simulink model "4_MERGED_STATES"  (R2020a)
settings: Solver=FixedStepAuto  StartTime=0.0  StopTime=10.0  FixedStep=1e-3  RelTol=1e-3  EnableMultiTasking=on
undefined symbols (not defined in the file): D0, D1, D10, D11, D12, D13, D2, D3, D4, D5, D6, D7, D8, D9, PTA0, PTA1, PTA2, PTB23, PTB9, PTC16, PTC17, PTC2, PTC3, PTC4, PTD0, PTD1, PTD2, PTD3
libraries: frdmk64flib x14
settings Model: ExtModeTrigDuration=5  Creator=marry  LastModifiedBy=amnay
settings OptimizationCC: EnhancedBackFolding=on  PassReuseOutputArgsAs=Individual arguments  ZeroExternalMemoryAtStartup=off  ZeroInternalMemoryAtStartup=off  MaxStackSize=64  OptimizeBlockOrder=speed  DifferentSizesBufferReuse=on  OptimizationCustomize=off  EfficientTunableParamExpr=on
settings DebuggingCC: ParameterTunabilityLossMsg=error
settings HardwareCC: ProdBitPerPointer=32  ProdBitPerSizeT=32  ProdBitPerPtrDiffT=32  ProdLargestAtomicInteger=Long  ProdLargestAtomicFloat=Double  ProdWordSize=32  ProdHWDeviceType=ARM Compatible->ARM Cortex
settings SFSimCC: MATLABDynamicMemAlloc=off
settings RTWCC: SystemTargetFile=ert.tlc  HardwareBoard=NXP FRDM-K64F  TemplateMakefile=ert_default_tmf  Toolchain=GNU Tools for ARM Embedded Processors
settings CodeAppCC: ForceParamTrailComments=on  IgnoreCustomStorageClasses=off  OperatorAnnotations=on  SimulinkDataObjDesc=on  SFDataObjDesc=on  InsertBlockDesc=on

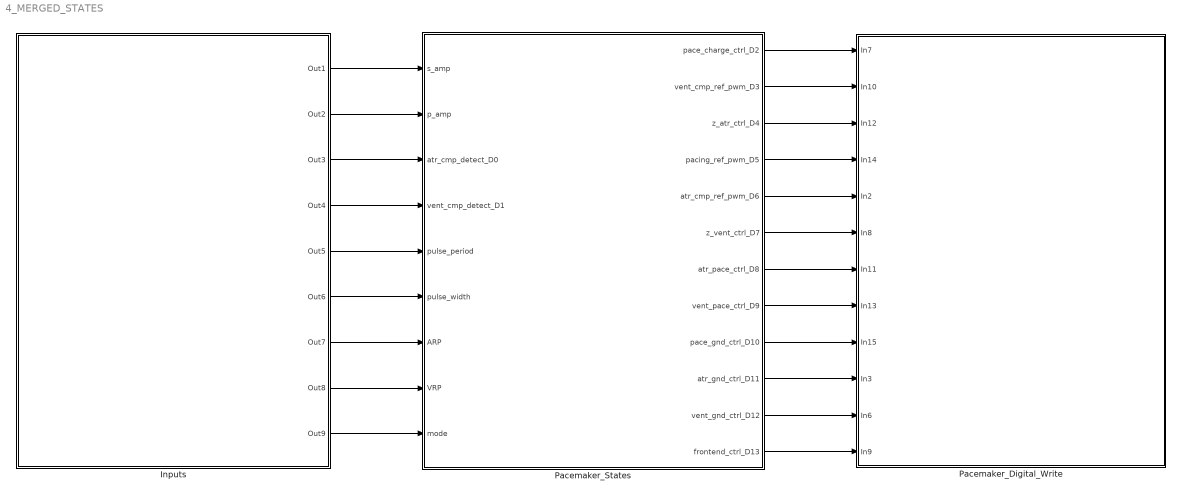
== system 4_MERGED_STATES ==
  Inputs : Subsystem
  Pacemaker_Digital_Write : Subsystem
  Pacemaker_States : Stateflow chart  TreatAsAtomicUnit=on
      settings: PortSchema="{\"entries\":[{\"content\":{\"sides\":[{\"content\":{\"connectorIds\":[\"In4\",\"In1\",\"In8\",\"In6\",\"In2\",\"In3\",\"In9\",\"In5\",\"In7\"]},\"type\":\"ConnectorPlacement.EquallySpacedRectSide\",\"uuid\":\"20680cc3-5670-44aa-8281-63eeb652eb93\"},{\"content\":{\"connectorIds\":[\"Out10\",\"Out7\",\"Out2\",\"Out8\",\"Out4\",\"Out1\",\"Out11\",\"Out3\",\"Out9\",\"Out5\",\"Out6\",\"Out12\"],\"side\":\"RIGHT\"},\"type\":\"ConnectorPlacement.EquallySpacedRectSide\",\"uuid\":\"3c751831-05e0-44c5-9153-358c656103ce\"},{\"content\":{\"connectorIds\":[],\"side\":\"TOP\"},\"type\":\"ConnectorPlacement.EquallySpacedRectSide\",\"uuid\":\"7efa84d7-9e28-4c8b-883e-bb8c609184af\"}]},\"type\":\"ConnectorPlacement.EquallySpacedConnector\",\"uuid\":\"9ce20c72-f6aa-4a08-b105-da4ff85e8db9\"}],\"packageUris\":[\"http://schema.mathworks.com/mf0/Connector/19700101\"],\"version\":\"1.0\"}"
  wires:
  Pacemaker_States/10(pace_charge_ctrl_D2) -> Pacemaker_Digital_Write/1(In7)
  Pacemaker_States/7(vent_cmp_ref_pwm_D3) -> Pacemaker_Digital_Write/2(In10)
  Pacemaker_States/8(pacing_ref_pwm_D5) -> Pacemaker_Digital_Write/4(In14)
  Pacemaker_States/2(z_atr_ctrl_D4) -> Pacemaker_Digital_Write/3(In12)
  Pacemaker_States/4(atr_cmp_ref_pwm_D6) -> Pacemaker_Digital_Write/5(In2)
  Pacemaker_States/1(z_vent_ctrl_D7) -> Pacemaker_Digital_Write/6(In8)
  Pacemaker_States/11(atr_pace_ctrl_D8) -> Pacemaker_Digital_Write/7(In11)
  Pacemaker_States/3(vent_pace_ctrl_D9) -> Pacemaker_Digital_Write/8(In13)
  Pacemaker_States/9(pace_gnd_ctrl_D10) -> Pacemaker_Digital_Write/9(In15)
  Pacemaker_States/5(atr_gnd_ctrl_D11) -> Pacemaker_Digital_Write/10(In3)
  Pacemaker_States/6(vent_gnd_ctrl_D12) -> Pacemaker_Digital_Write/11(In6)
  Pacemaker_States/12(frontend_ctrl_D13) -> Pacemaker_Digital_Write/12(In9)
  Inputs/1(Out1) -> Pacemaker_States/4(s_amp)
  Inputs/2(Out2) -> Pacemaker_States/1(p_amp)
  Inputs/3(Out3) -> Pacemaker_States/8(atr_cmp_detect_D0)
  Inputs/4(Out4) -> Pacemaker_States/6(vent_cmp_detect_D1)
  Inputs/5(Out5) -> Pacemaker_States/2(pulse_period)
  Inputs/6(Out6) -> Pacemaker_States/3(pulse_width)
  Inputs/7(Out7) -> Pacemaker_States/9(ARP)
  Inputs/8(Out8) -> Pacemaker_States/5(VRP)
  Inputs/9(Out9) -> Pacemaker_States/7(mode)

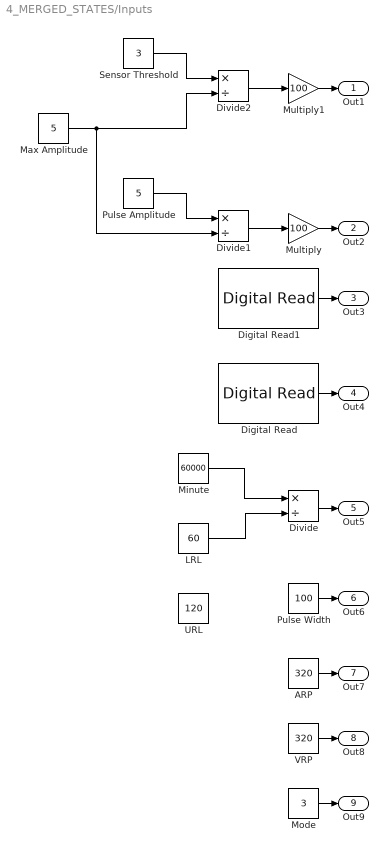
== system 4_MERGED_STATES/Inputs ==
  ARP : Constant  Value=320
  Digital Read : frdmk64flib/Digital Read  Whichpin=PTC17 (D1)  SampleTime=-1
  Digital Read1 : frdmk64flib/Digital Read  Whichpin=PTC16 (D0)  SampleTime=-1
  Divide : Product  Inputs=*/
  Divide1 : Product  Inputs=*/
  Divide2 : Product  Inputs=*/
  LRL : Constant  Value=60
  Max Amplitude : Constant  Value=5
  Minute : Constant  Value=60000
  Mode : Constant  Value=3
  Multiply : Gain  Gain=100
  Multiply1 : Gain  Gain=100
  Pulse Amplitude : Constant  Value=5
  Pulse Width : Constant  Value=100
  Sensor Threshold : Constant  Value=3
  URL : Constant  Value=120
  VRP : Constant  Value=320
  Out1 : Outport
  Out2 : Outport  Port=2
  Out3 : Outport  Port=3
  Out4 : Outport  Port=4
  Out5 : Outport  Port=5
  Out6 : Outport  Port=6
  Out7 : Outport  Port=7
  Out8 : Outport  Port=8
  Out9 : Outport  Port=9
  wires:
  VRP/1 -> Out8/1
  Sensor Threshold/1 -> Divide2/1
  Max Amplitude/1 -> Divide2/2, Divide1/2
  Pulse Amplitude/1 -> Divide1/1
  Minute/1 -> Divide/1
  Divide1/1 -> Multiply/1
  LRL/1 -> Divide/2
  Divide2/1 -> Multiply1/1
  ARP/1 -> Out7/1
  Digital Read1/1 -> Out3/1
  Multiply1/1 -> Out1/1
  Digital Read/1 -> Out4/1
  Divide/1 -> Out5/1
  Multiply/1 -> Out2/1
  Pulse Width/1 -> Out6/1
  Mode/1 -> Out9/1

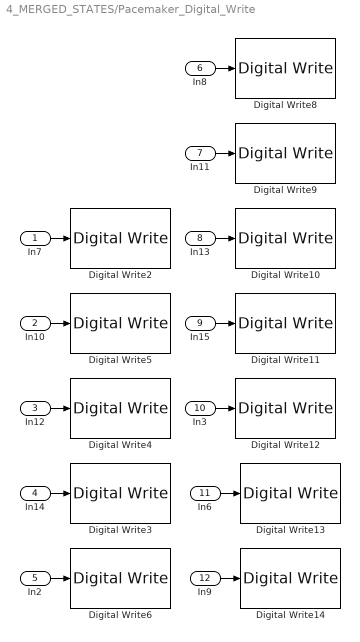
== system 4_MERGED_STATES/Pacemaker_Digital_Write ==
  In7 : Inport
  In10 : Inport  Port=2
  In12 : Inport  Port=3
  In14 : Inport  Port=4
  In2 : Inport  Port=5
  In8 : Inport  Port=6
  In11 : Inport  Port=7
  In13 : Inport  Port=8
  In15 : Inport  Port=9
  In3 : Inport  Port=10
  In6 : Inport  Port=11
  In9 : Inport  Port=12
  Digital Write10 : frdmk64flib/Digital Write  Whichpin=PTC4 (D9)
  Digital Write11 : frdmk64flib/Digital Write  Whichpin=PTD0 (D10)
  Digital Write12 : frdmk64flib/Digital Write  Whichpin=PTD2 (D11)
  Digital Write13 : frdmk64flib/Digital Write  Whichpin=PTD3 (D12)
  Digital Write14 : frdmk64flib/Digital Write  Whichpin=PTD1 (D13)
  Digital Write2 : frdmk64flib/Digital Write  Whichpin=PTB9 (D2)
  Digital Write3 : frdmk64flib/Digital Write  Whichpin=PTA2 (D5)
  Digital Write4 : frdmk64flib/Digital Write  Whichpin=PTB23 (D4)
  Digital Write5 : frdmk64flib/Digital Write  Whichpin=PTA1 (D3)
  Digital Write6 : frdmk64flib/Digital Write  Whichpin=PTC2 (D6)
  Digital Write8 : frdmk64flib/Digital Write  Whichpin=PTC3 (D7)
  Digital Write9 : frdmk64flib/Digital Write  Whichpin=PTA0 (D8)
  wires:
  In15/1 -> Digital Write11/1
  In12/1 -> Digital Write4/1
  In13/1 -> Digital Write10/1
  In7/1 -> Digital Write2/1
  In14/1 -> Digital Write3/1
  In8/1 -> Digital Write8/1
  In6/1 -> Digital Write13/1
  In11/1 -> Digital Write9/1
  In2/1 -> Digital Write6/1
  In3/1 -> Digital Write12/1
  In9/1 -> Digital Write14/1
  In10/1 -> Digital Write5/1

== stateflow chart 4_MERGED_STATES/Pacemaker_States ==
  state VOO_State
    state Charging
      entry:
      pacing_ref_pwm_D5 = p_amp;
      pace_charge_ctrl_D2 = 1;
      vent_pace_ctrl_D9 = 0;
      vent_gnd_ctrl_D12 = 1;
      pace_gnd_ctrl_D10 = 0;
      z_vent_ctrl_D7 = 0;
    state Pacing
      entry:
      pace_charge_ctrl_D2 = 0;
      vent_pace_ctrl_D9 = 1;
      vent_gnd_ctrl_D12 = 0;
      pace_gnd_ctrl_D10 = 1;
    (default) -> VOO_State.Charging
    VOO_State.Charging -> VOO_State.Pacing : [after(pulse_period - pulse_width,msec)]
    VOO_State.Pacing -> VOO_State.Charging : [after(pulse_width,msec)]
  state AAI_State
    state AAI_Charging_Sensing
      entry:
      frontend_ctrl_D13= 1;
      pacing_ref_pwm_D5= p_amp;
      atr_cmp_ref_pwm_D6= s_amp;
      pace_charge_ctrl_D2 = 1;
      atr_pace_ctrl_D8 = 0;
      atr_gnd_ctrl_D11= 1;
      pace_gnd_ctrl_D10= 1;
      z_atr_ctrl_D4= 0;
    state AAI_Pacing
      entry:
      frontend_ctrl_D13= 0;
      pace_charge_ctrl_D2 = 0;
      pace_gnd_ctrl_D10 = 1;
      atr_pace_ctrl_D8 = 1;
      atr_gnd_ctrl_D11= 0;
      z_atr_ctrl_D4= 0;
      pacing_ref_pwm_D5= p_amp;
    (junction 82) -> AAI_Charging_Sensing [order 1] : [atr_cmp_detect_D0 == 1]
    (default) -> AAI_Charging_Sensing
    AAI_Charging_Sensing -> (junction 82) : [after(ARP-pulse_width,msec)]
    (junction 82) -> AAI_Pacing [order 2] : after(pulse_period- ARP,msec)
    AAI_Pacing -> AAI_Charging_Sensing : [after(pulse_width,msec)]
  state AOO_State
    state Charging
      % Initial state - charging the capacitor
      entry:
      pacing_ref_pwm_D5= p_amp;
      pace_charge_ctrl_D2 = 1;
      atr_pace_ctrl_D8 = 0;
      atr_gnd_ctrl_D11= 1;
      pace_gnd_ctrl_D10= 0;
      z_atr_ctrl_D4= 0;
    state Pacing
      entry:
      pace_charge_ctrl_D2 = 0;
      atr_pace_ctrl_D8 = 1;
      atr_gnd_ctrl_D11= 0;
      pace_gnd_ctrl_D10 = 1;
    (default) -> AOO_State.Charging
    AOO_State.Charging -> AOO_State.Pacing : [after(pulse_period - pulse_width,msec)]
    AOO_State.Pacing -> AOO_State.Charging : [after(pulse_width,msec)]
  state Start_State
  state VVI_State
    state Pacing
      entry:
      frontend_ctrl_D13 = 0;
      pace_charge_ctrl_D2 = 0;
      vent_pace_ctrl_D9 = 1;
      vent_gnd_ctrl_D12 = 0;
      pace_gnd_ctrl_D10 = 1;
      pacing_ref_pwm_D5 = p_amp;
    state Charge_and_Sense
      entry:
      frontend_ctrl_D13 = 1;
      pacing_ref_pwm_D5 = p_amp;
      vent_cmp_ref_pwm_D3 = s_amp;
      pace_charge_ctrl_D2 = 1;
      vent_pace_ctrl_D9 = 0;
      vent_gnd_ctrl_D12 = 1;
      pace_gnd_ctrl_D10 = 1;
      z_vent_ctrl_D7 = 0;
    (junction 33) -> Charge_and_Sense [order 1] : [vent_cmp_detect_D1 == 1]
    (default) -> Charge_and_Sense
    Charge_and_Sense -> (junction 33) : [after(VRP-pulse_width,msec)]
    (junction 33) -> VVI_State.Pacing [order 2] : after(pulse_period- VRP,msec)
    VVI_State.Pacing -> Charge_and_Sense : [after(pulse_width,msec)]
  Start_State -> VOO_State [order 2] : [mode == 2]
  VOO_State -> Start_State : [mode ~= 2]
  (default) -> Start_State
  AAI_State -> Start_State : [mode ~= 3]
  Start_State -> AOO_State [order 1] : [mode == 1]
  Start_State -> AAI_State [order 4] : [mode == 3]
  AOO_State -> Start_State : [mode ~= 1]
  Start_State -> VVI_State [order 3] : [mode == 4]
  VVI_State -> Start_State : [mode ~= 4]
  data: p_amp input; pulse_period input; pulse_width input; s_amp input; VRP input; z_vent_ctrl_D7 output; z_atr_ctrl_D4 output; vent_pace_ctrl_D9 output; atr_cmp_ref_pwm_D6 output; atr_gnd_ctrl_D11 output; vent_gnd_ctrl_D12 output; vent_cmp_ref_pwm_D3 output; pacing_ref_pwm_D5 output; pace_gnd_ctrl_D10 output; pace_charge_ctrl_D2 output; atr_pace_ctrl_D8 output; frontend_ctrl_D13 output; vent_cmp_detect_D1 input; mode input; atr_cmp_detect_D0 input; ARP input
